simulink model "Controllo_inseguimento_uniciclo"  (R2021b)
settings: Solver=ode1be  StartTime=0.0  StopTime=20  FixedStep=1e-3  RelTol=1e-3
values from neighbouring files (symbols this model uses):
  kl = [l1 l2 k]    [init.m]
  q0 = [-10; 5; pi/2]    [init.m]
  q0_hat = [40; -5; pi]    [init.m]
  v_hat = 10    [init.m]
  w_hat = 1    [init.m]
settings Model: Creator=vince  LastModifiedBy=vince

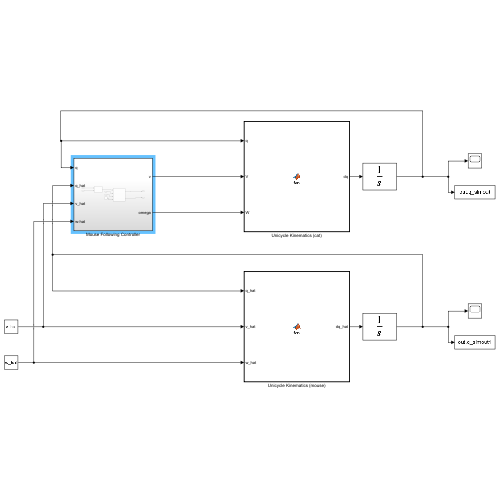
[thumbnail: Simulink's stored preview of the top-level diagram]
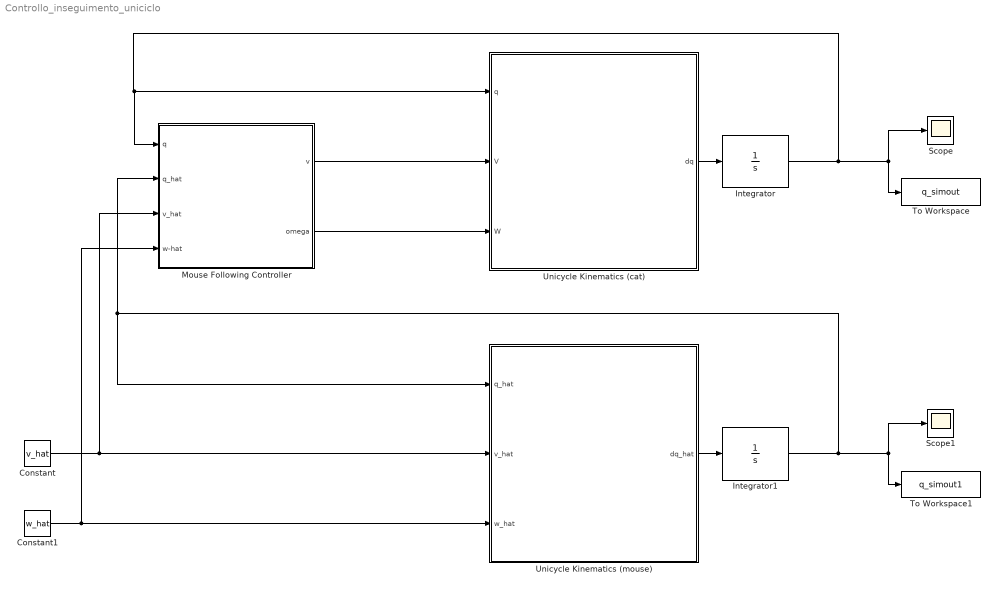
== system Controllo_inseguimento_uniciclo ==
  Constant : Constant  Value=v_hat
  Constant1 : Constant  Value=w_hat
  Integrator : Integrator  InitialCondition=q0
  Integrator1 : Integrator  InitialCondition=q0_hat
  Mouse Following Controller : Subsystem
  Scope : Scope
  Scope1 : Scope
  To Workspace : ToWorkspace  VariableName=q_simout  SaveFormat=Timeseries  SampleTime=-1
  To Workspace1 : ToWorkspace  VariableName=q_simout1  SaveFormat=Timeseries  SampleTime=-1
  Unicycle Kinematics (cat) : MATLAB Function  TreatAsAtomicUnit=on
  Unicycle Kinematics (mouse) : MATLAB Function  TreatAsAtomicUnit=on
  wires:
  Integrator/1 -> Mouse Following Controller/1(q), Unicycle Kinematics (cat)/1(q), Scope/1, To Workspace/1
  Unicycle Kinematics (cat)/1(dq) -> Integrator/1
  Mouse Following Controller/1(v) -> Unicycle Kinematics (cat)/2(V)
  Mouse Following Controller/2(omega) -> Unicycle Kinematics (cat)/3(W)
  Unicycle Kinematics (mouse)/1(dq_hat) -> Integrator1/1
  Constant/1 -> Unicycle Kinematics (mouse)/2(v_hat), Mouse Following Controller/3(v_hat)
  Constant1/1 -> Unicycle Kinematics (mouse)/3(w_hat), Mouse Following Controller/4(w-hat)
  Integrator1/1 -> Mouse Following Controller/2(q_hat), Unicycle Kinematics (mouse)/1(q_hat), To Workspace1/1, Scope1/1

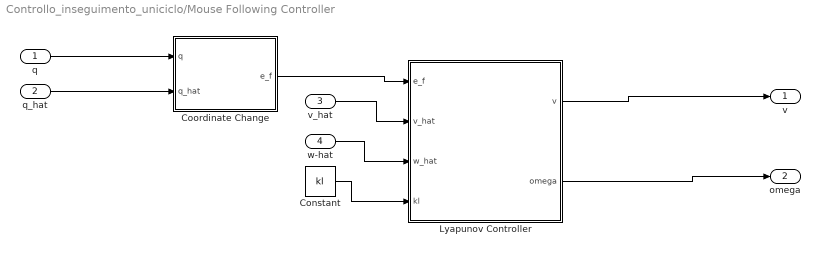
== system Controllo_inseguimento_uniciclo/Mouse Following Controller ==
  q : Inport
  q_hat : Inport  Port=2
  v_hat : Inport  Port=3
  w-hat : Inport  Port=4
  Constant : Constant  Value=kl
  Coordinate Change : MATLAB Function  TreatAsAtomicUnit=on
  Lyapunov Controller : MATLAB Function  TreatAsAtomicUnit=on
  v : Outport
  omega : Outport  Port=2
  wires:
  Lyapunov Controller/1(v) -> v/1
  Lyapunov Controller/2(omega) -> omega/1
  Coordinate Change/1(e_f) -> Lyapunov Controller/1(e_f)
  Constant/1 -> Lyapunov Controller/4(kl)
  w-hat/1 -> Lyapunov Controller/3(w_hat)
  v_hat/1 -> Lyapunov Controller/2(v_hat)
  q/1 -> Coordinate Change/1(q)
  q_hat/1 -> Coordinate Change/2(q_hat)

== matlab function Controllo_inseguimento_uniciclo/Mouse Following Controller/Lyapunov Controller ==
  data: e_f input; v output; v_hat input; omega output; w_hat input; kl input
function [v, omega] = fcn(e_f, v_hat, w_hat, kl)

l1 = kl(1); 
l2 = kl(2); 
k = kl(3);

% control
v = v_hat*cos(e_f(3)) - l1*e_f(1);

% se x tende a 0 allora sen(x)/x = 1
omega = w_hat - e_f(2)*v_hat/k - l2*sin(e_f(3));

== matlab function Controllo_inseguimento_uniciclo/Unicycle Kinematics (mouse) ==
  data: q_hat input; dq_hat output; v_hat input; w_hat input
function dq_hat = fcn(q_hat, v_hat, w_hat)

x = q_hat(1); y = q_hat(2); th = q_hat(3);

dx = v_hat * cos(th);
dy = v_hat * sin(th);
dth = w_hat;

dq_hat = [dx; dy; dth];

== matlab function Controllo_inseguimento_uniciclo/Unicycle Kinematics (cat) ==
  data: q input; dq output; V input; W input
function dq = fcn(q, V, W)

x = q(1); y = q(2); th = q(3);

dx = V * cos(th);
dy = V * sin(th);
dth = W;

dq = [dx; dy; dth];

== matlab function Controllo_inseguimento_uniciclo/Mouse Following Controller/Coordinate Change ==
  data: e_f output; q input; q_hat input
function e_f = fcn(q, q_hat)

%coordinate inseguitore (cat)
x = q(1); y = q(2); th = q(3);

%coordinate inseguito (mouse)
x_hat = q_hat(1); y_hat = q_hat(2); th_hat = q_hat(3);

%definisco l'errore nella terna mondo 
e = [x-x_hat; y-y_hat; 0];

%definisco una matrice di cambio di coordinate

t_f = [ cos(th), sin(th), -x*cos(th)-y*sin(th); -sin(th), cos(th), x*sin(th)-y*cos(th); 0, 0, 1]; 

%mi porto nel sistema di riferimento coincidente con l'inseguitore così da
%minimizzare poi l'errore tra il gatto e il topo
e_f = t_f*e;
e_f(3) = th-th_hat;
